simulink model "Lab2Part3b"  (R2022a)
settings: Solver=VariableStepAuto  StartTime=0.0  StopTime=2  RelTol=1e-3
settings Model: Creator=gitan  LastModifiedBy=yooncha5
settings DebuggingCC: UnconnectedInputMsg=warning  UnconnectedOutputMsg=warning  UnconnectedLineMsg=warning
settings RTWCC: DLArmComputeVersion=19.05

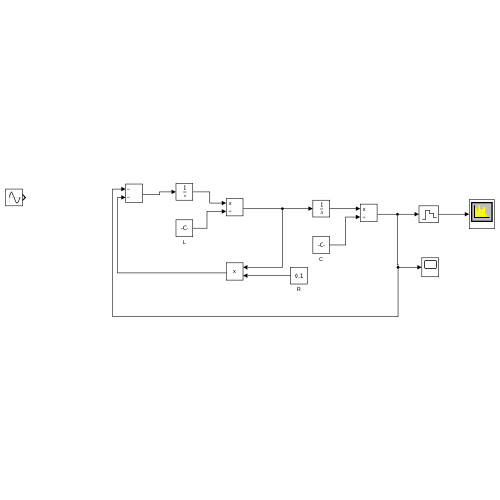
[thumbnail: Simulink's stored preview of the top-level diagram]
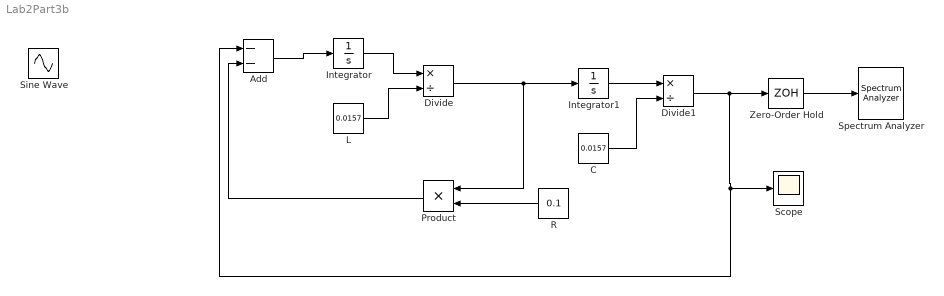
== system Lab2Part3b ==
  Add : Sum  Inputs=--
  C : Constant  Value=0.0157
  Divide : Product  Inputs=*/
  Divide1 : Product  Inputs=*/
  Integrator : Integrator
  Integrator1 : Integrator
  L : Constant  Value=0.0157
  Product : Product
  R : Constant  Value=0.1
  Scope : Scope
  Sine Wave : Sin  Amplitude=4/3.14159  Frequency=32*2*3.14  SampleTime=0
  Spectrum Analyzer : SpectrumAnalyzer
  Zero-Order Hold : ZeroOrderHold  SampleTime=1/1024
  wires:
  C/1 -> Divide1/2
  R/1 -> Product/2
  Divide1/1 -> Add/1, Scope/1, Zero-Order Hold/1
  Add/1 -> Integrator/1
  Divide/1 -> Product/1, Integrator1/1
  Integrator1/1 -> Divide1/1
  Integrator/1 -> Divide/1
  Zero-Order Hold/1 -> Spectrum Analyzer/1
  L/1 -> Divide/2
  Product/1 -> Add/2
